simulink model "importTreeBagger_3004"  (R2017a)
settings: Solver=FixedStepAuto  StartTime=0.0  StopTime=simTime  FixedStep=Dt  RelTol=1e-3  EnableMultiTasking=on
values from neighbouring files (symbols this model uses):
  D0 = 35.783396242    [cic2017_fase1_boiler.mat]    (also in compare_rf_boiler.m = 35.7834; control_Caldera_3004.m = 35.7834; mpcGASimulink_2205_dummy.m = 35.7834; mpc_design_parameters_0206.mat = 35.7834)
  U0 = [32.9815865199 46.2282063472 25.3416381967]    [cic2017_fase1_boiler.mat]    (also in compare_rf_boiler.m = [32.9816   46.2282   25.3416]; control_Caldera_3004.m = [32.9816   46.2282   25.3416]; mpcGASimulink_2205_dummy.m = [32.9816   46.2282   25.3416]; mpc_design_parameters_0206.mat = [32.9816 46.2282 25.3416])
  Y0 = [41.4119839556 28.7552838432 38.6036799989]    [cic2017_fase1_boiler.mat]    (also in compare_rf_boiler.m = [41.4120   28.7553   38.6037]; control_Caldera_3004.m = [41.4120   28.7553   38.6037]; mpcGASimulink_2205_dummy.m = [41.4120   28.7553   38.6037]; mpc_design_parameters_0206.mat = [41.412 28.7553 38.6037])
libraries: mpclib x1
settings Model: Creator=Pablo Diaz  LastModifiedBy=Pablo Diaz
settings OptimizationCC: LifeSpan=inf
settings DebuggingCC: SFUnexpectedBacktrackingDiag=warning  SFNoUnconditionalDefaultTransitionDiag=warning  SFExecutionAtInitializationDiag=none
settings GRTTargetCC: TargetLangStandard=C89/C90 (ANSI)
settings ConfigComp: CovMetricSettings=dw  CovHtmlReporting=on  CovSaveCumulativeToWorkspaceVar=on  CovSaveSingleToWorkspaceVar=on  CovExternalEMLEnable=off

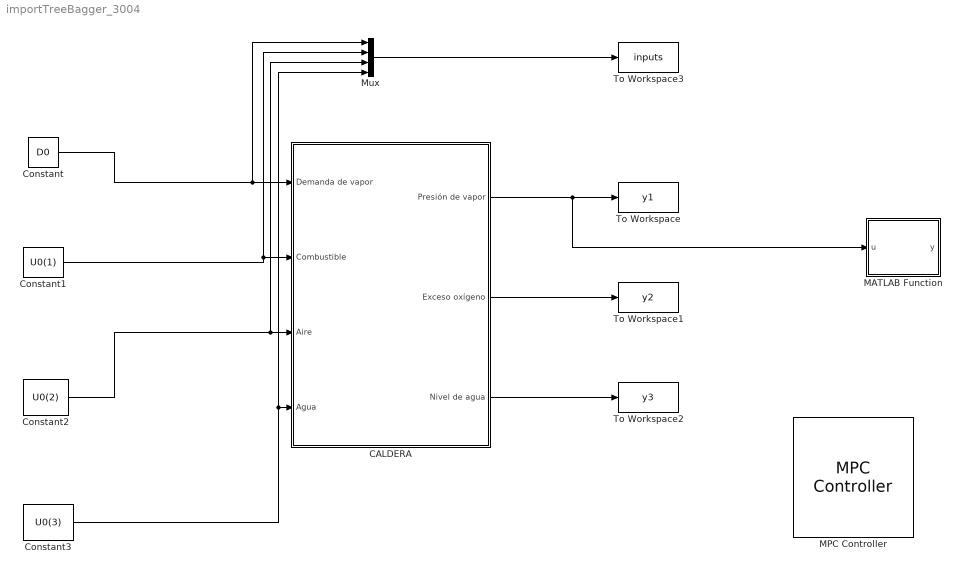
== system importTreeBagger_3004 ==
  CALDERA : Subsystem
  Constant : Constant  Value=D0
  Constant1 : Constant  Value=U0(1)
  Constant2 : Constant  Value=U0(2)
  Constant3 : Constant  Value=U0(3)
  MATLAB Function : MATLAB Function  TreatAsAtomicUnit=on
  MPC Controller : mpclib/MPC Controller  SCDEnableBlockLinearizationSpecification=on  is_multiple=0  enable_value=0  return_u0=off  ref_from_ws=off  ref_signal_name=[]  ref_preview=off  md_from_ws=off  md_signal_name=[]  md_preview=off  from_project=off  project_file=MPCtask.mat  md_inport=on  mv_inport=off  cost_outport=off  return_sequence=off  return_qpstatus=off  return_state=off  state_inport=off  lims_inport=off  ywt_inport=off  is_designfromscratch=0  uwt_inport=off  duwt_inport=off  rhoeps_inport=off  uref_inport=off  n_ts=1  n_mv=1  n_md=1  n_ud=0  n_mo=1  n_uo=0  BlockDataType=double  SampleTimeInherited=off  switch_inport=off
  Mux : Mux
  To Workspace : ToWorkspace  VariableName=y1  SaveFormat=Structure With Time  SampleTime=-1
  To Workspace1 : ToWorkspace  VariableName=y2  SaveFormat=Structure With Time  SampleTime=-1
  To Workspace2 : ToWorkspace  VariableName=y3  SaveFormat=Structure With Time  SampleTime=-1
  To Workspace3 : ToWorkspace  VariableName=inputs  SaveFormat=Structure With Time  SampleTime=-1
  wires:
  CALDERA/2(Exceso oxígeno) -> To Workspace1/1
  CALDERA/3(Nivel de agua) -> To Workspace2/1
  Constant2/1 -> Mux/3, CALDERA/3(Aire)
  Constant3/1 -> Mux/4, CALDERA/4(Agua)
  Constant1/1 -> Mux/2, CALDERA/2(Combustible)
  Constant/1 -> Mux/1, CALDERA/1(Demanda de vapor)
  Mux/1 -> To Workspace3/1
  CALDERA/1(Presión de vapor) -> MATLAB Function/1(u), To Workspace/1

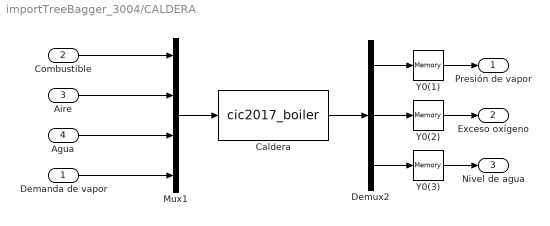
== system importTreeBagger_3004/CALDERA ==
  Demanda de vapor : Inport
  Combustible : Inport  Port=2
  Aire : Inport  Port=3
  Agua : Inport  Port=4
  Caldera : S-Function  FunctionName=cic2017_boiler  Parameters=Y0,[U0 D0]  SFunctionDeploymentMode=off  EnableBusSupport=off
  Demux2 : Demux  Outputs=3
  Mux1 : Mux
  Y0(1) : Memory  X0=Y0(1)
  Y0(2) : Memory  X0=Y0(2)
  Y0(3) : Memory  X0=Y0(3)
  Presión de vapor : Outport
  Exceso oxígeno : Outport  Port=2
  Nivel de agua : Outport  Port=3
  wires:
  Caldera/1 -> Demux2/1
  Aire/1 -> Mux1/2
  Agua/1 -> Mux1/3
  Demanda de vapor/1 -> Mux1/4
  Combustible/1 -> Mux1/1
  Mux1/1 -> Caldera/1
  Demux2/1 -> Y0(1)/1
  Demux2/2 -> Y0(2)/1
  Demux2/3 -> Y0(3)/1
  Y0(1)/1 -> Presión de vapor/1
  Y0(2)/1 -> Exceso oxígeno/1
  Y0(3)/1 -> Nivel de agua/1

== matlab function importTreeBagger_3004/MATLAB Function ==
  data: u input; y output; RF parameter
function y = fcn(u,RF)
% coder.extrinsic('importRF');
% y = coder.nullcopy(zeros(1));
% caca = importRF();
% caca = 10;
caca = RF.a;
y = caca*u;
